simulink model "LineAnalyser"  (R2015b)
settings: Solver=VariableStepAuto  StartTime=0.0  StopTime=10.0  RelTol=1e-3
values from neighbouring files (symbols this model uses):
  Rad2Deg = 180/pi    (= 57.2956455309)    [ControlInit.m]
undefined symbols (not defined in the file or in its folder): Imag, Real
libraries: powerlib x9
settings Model: Creator=Emilio  LastModifiedBy=Emilio

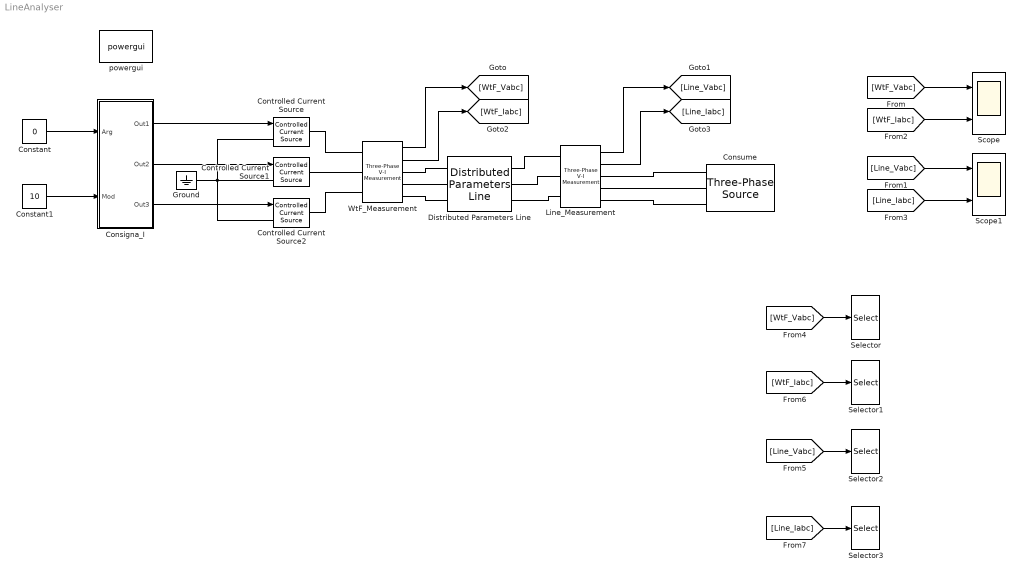
== system LineAnalyser ==
  Consigna_I : Subsystem
  Constant : Constant  Value=0
  Constant1 : Constant  Value=10
  Consume : powerlib/Electrical Sources/Three-Phase Source  InternalConnection=Yg  VoltagePhases=off  Voltage=220e3  PhaseAngle=0  Voltage_phases=[25e3 25e3 25e3]/sqrt(3)  PhaseAngles_phases=[0 -120 +120]  Frequency=50  NonIdealSource=on  SpecifyImpedance=off  Resistance=0.8929  Inductance=16.58e-3  ShortCircuitLevel=100e6  BaseVoltage=25e3  XRratio=7  BusType=swing  Pref=10e3  Qref=0  Prefabc=[10e3, 10e3, 10e3]  Qrefabc=[0, 0, 0]  Qmin=-inf  Qmax=inf
  Controlled Current Source : powerlib/Electrical Sources/Controlled Current Source  Initialize=off  Source_Type=AC  Amplitude=0  Phase=0  Frequency=0  Measurements=None
  Controlled Current Source1 : powerlib/Electrical Sources/Controlled Current Source  Initialize=off  Source_Type=AC  Amplitude=0  Phase=0  Frequency=0  Measurements=None
  Controlled Current Source2 : powerlib/Electrical Sources/Controlled Current Source  Initialize=off  Source_Type=AC  Amplitude=0  Phase=0  Frequency=0  Measurements=None
  Distributed Parameters Line : powerlib/Elements/Distributed Parameters Line  Phases=3  Frequency=60  Resistance=[0.01273 0.3864]  Inductance="[0.9337e-3  4.1264e-3]"  Capacitance=[12.74e-9 7.751e-9]  Length=100  x1=[1.35206107618783e-11 25200.2128645645 25200.2128645645;314.159265358979 314.159265358979 314.159265358979;2.22610747025198 0.414630755481806 -1.15616557131309]  x2=[9.09494701772928e-12 25052.4300261818 25052.4300261818;314.159265358979 314.159265358979 314.159265358979;0.465830985575936 0.414886509193973 -1.15590981760092]  x3=[2.22429603843386e-13 92.7585410401311 92.758541040131;314.159265358979 314.159265358979 314.159265358979;-1.48085014522748 0.414630755481802 -1.15616557131309]  x4=[2.03633313157801e-13 92.7579023126405 92.7579023126408;314.159265358979 314.159265358979 314.159265358979;1.56386141505283 0.306405550476882 -1.26439077631802]  x5=0.000565541566995742  V1=ones(3,3)  V2=ones(3,3)  I1=ones(3,3)  I2=ones(3,3)  nHarmo=1  Measurements=None
  Ground : powerlib/Elements/Ground  LConnTagsString=a
  Line_Measurement : powerlib/Measurements/Three-Phase V-I Measurement  VoltageMeasurement=phase-to-ground  SetLabelV=off  LabelV=WtF_Vabc  Vpu=off  VpuLL=off  CurrentMeasurement=yes  SetLabelI=off  LabelI=WtF_Iabc  Ipu=off  Pbase=100e6  Vbase=500e3  OutputType=Real-Imag  PhasorSimulation=on  PSBequivalent=0
  Scope : Scope  NumInputPorts=2
  Scope1 : Scope  NumInputPorts=2
  Selector{,1..3} (4 alike) : Selector  InputPortWidth=6  IndexOptions=Index vector (dialog)  Indices=[1 4]  OutputSizes=1
  WtF_Measurement : powerlib/Measurements/Three-Phase V-I Measurement  VoltageMeasurement=phase-to-ground  SetLabelV=off  LabelV=WtF_Vabc  Vpu=off  VpuLL=off  CurrentMeasurement=yes  SetLabelI=off  LabelI=WtF_Iabc  Ipu=off  Pbase=100e6  Vbase=500e3  OutputType=Real-Imag  PhasorSimulation=on  PSBequivalent=0
  powergui : powerlib/powergui  Priority=1  SimulationMode=Phasor  SolverType=Tustin/Backward Euler (TBE)  SampleTime=50e-6  frequency=50  SPID=off  DisableSnubberDevices=off  DisableRonSwitches=off  DisableVfSwitches=off  SwTol=0  DisplayEquations=off  Interpol=off  ExternalGateDelay=off  methode=off  Ts=10  FunctionMessages=off  echomessages=off  HookPort=off  EnableUseOfTLC=off  x0status=blocks  frequencyindice=50  Pbase=100e6  ErrMax=1e-4  Iterations=50  UnitsV=kV  UnitsW=MW  buscounter=0  RestoreLinks=warning  ResistiveCurrentMeasurement=off  Frange=[0:2:500]  Ylog=off  Xlog=on  ShowGrid=off  save=off  variable=ZData  structure=0  ZoomFFT=off  StartTime=0.0  cycles=1  DisplayStyle=1  fundamental=60  FreqAxis=off  MaxFrequency=1000  frequencyindicesteady=1  RmsSteady=1  display=off
  wires:
  Consigna_I/1(Out1) -> Controlled Current Source/1
  Consigna_I/2(Out2) -> Controlled Current Source1/1
  Consigna_I/3(Out3) -> Controlled Current Source2/1
  WtF_Measurement/1 -> [WtF_Vabc]
  Line_Measurement/1 -> [Line_Vabc]
  WtF_Measurement/2 -> [WtF_Iabc]
  Line_Measurement/2 -> [Line_Iabc]
  Constant/1 -> Consigna_I/1(Arg)
  Constant1/1 -> Consigna_I/2(Mod)
  [WtF_Vabc] -> Scope/1
  [WtF_Iabc] -> Scope/2
  [Line_Iabc] -> Scope1/2
  [Line_Vabc] -> Scope1/1
  [WtF_Vabc] -> Selector/1
  [WtF_Iabc] -> Selector1/1
  [Line_Vabc] -> Selector2/1
  [Line_Iabc] -> Selector3/1
  connections:
  Controlled Current Source2/LConn1 -- Controlled Current Source1/LConn1 -- Controlled Current Source/LConn1 -- Ground/LConn1
  WtF_Measurement/LConn3 -- Controlled Current Source2/RConn1
  WtF_Measurement/LConn2 -- Controlled Current Source1/RConn1
  WtF_Measurement/LConn1 -- Controlled Current Source/RConn1
  Distributed Parameters Line/LConn2 -- WtF_Measurement/RConn2
  WtF_Measurement/RConn1 -- Distributed Parameters Line/LConn1
  WtF_Measurement/RConn3 -- Distributed Parameters Line/LConn3
  Line_Measurement/LConn3 -- Distributed Parameters Line/RConn3
  Distributed Parameters Line/RConn2 -- Line_Measurement/LConn2
  Distributed Parameters Line/RConn1 -- Line_Measurement/LConn1
  Line_Measurement/RConn1 -- Consume/RConn3
  Line_Measurement/RConn2 -- Consume/RConn2
  Line_Measurement/RConn3 -- Consume/RConn1

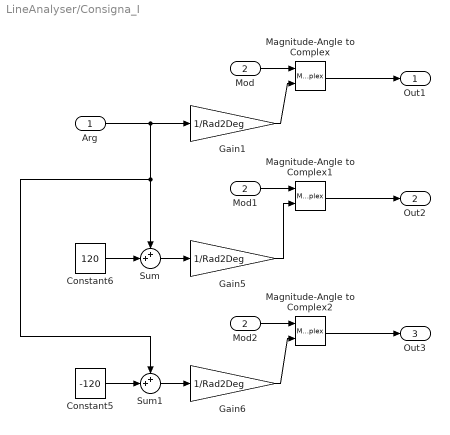
== system LineAnalyser/Consigna_I ==
  Arg : Inport
  Mod : Inport  Port=2
  Constant5 : Constant  Value=-120
  Constant6 : Constant  Value=120
  Gain1 : Gain  Gain=1/Rad2Deg
  Gain5 : Gain  Gain=1/Rad2Deg
  Gain6 : Gain  Gain=1/Rad2Deg
  Magnitude-Angle to Complex : MagnitudeAngleToComplex
  Magnitude-Angle to Complex1 : MagnitudeAngleToComplex
  Magnitude-Angle to Complex2 : MagnitudeAngleToComplex
  Mod1 : InportShadow  Port=2
  Mod2 : InportShadow  Port=2
  Sum : Sum  Inputs=++|
  Sum1 : Sum  Inputs=++|
  Out1 : Outport
  Out2 : Outport  Port=2
  Out3 : Outport  Port=3
  wires:
  Magnitude-Angle to Complex/1 -> Out1/1
  Magnitude-Angle to Complex1/1 -> Out2/1
  Magnitude-Angle to Complex2/1 -> Out3/1
  Gain5/1 -> Magnitude-Angle to Complex1/2
  Gain6/1 -> Magnitude-Angle to Complex2/2
  Mod2/1 -> Magnitude-Angle to Complex2/1
  Mod1/1 -> Magnitude-Angle to Complex1/1
  Mod/1 -> Magnitude-Angle to Complex/1
  Arg/1 -> Gain1/1, Sum/1, Sum1/1
  Sum1/1 -> Gain6/1
  Constant5/1 -> Sum1/2
  Sum/1 -> Gain5/1
  Constant6/1 -> Sum/2
  Gain1/1 -> Magnitude-Angle to Complex/2
